simulink model "ex5"  (R2021a)
settings: Solver=VariableStepAuto  StartTime=0.0  StopTime=120  RelTol=1e-7
values from neighbouring files (symbols this model uses):
  a = m*g*l/I    (= 1.96)    [aae666_hw8_ex5.m]
  b = 1/I    (= 0.1)    [aae666_hw8_ex5.m]
  K = [kp kd]    [aae666_hw8_ex5.m]
settings Model: Creator=Tomo  LastModifiedBy=Tomo

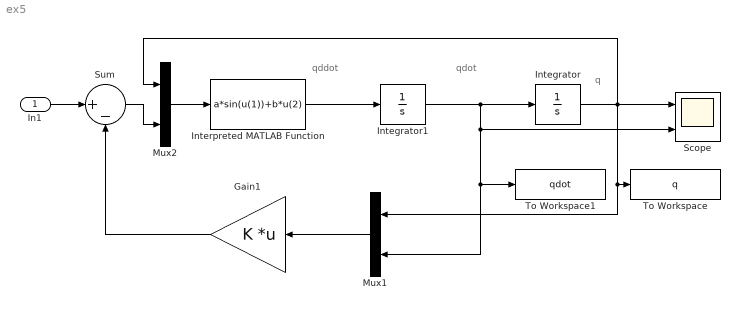
== system ex5 ==
  note: qddot
  note: qdot
  note: q
  In1 : Inport
  Gain1 : Gain  Gain=K  Multiplication=Matrix(K*u)
  Integrator : Integrator  InitialCondition=1
  Integrator1 : Integrator
  Interpreted MATLAB Function : MATLABFcn  MATLABFcn=a*sin(u(1))+b*u(2)
  Mux1 : Mux  Inputs=2
  Mux2 : Mux  Inputs=2
  Scope : Scope  NumInputPorts=2
  Sum : Sum  Inputs=|+-
  To Workspace : ToWorkspace  VariableName=q  SaveFormat=Structure With Time  SampleTime=-1
  To Workspace1 : ToWorkspace  VariableName=qdot  SaveFormat=Structure With Time  SampleTime=-1
  wires:
  Integrator1/1 -> To Workspace1/1, Mux1/2, Scope/2, Integrator/1
  Interpreted MATLAB Function/1 -> Integrator1/1
  Integrator/1 -> Mux2/1, To Workspace/1, Mux1/1, Scope/1
  Gain1/1 -> Sum/2
  Mux1/1 -> Gain1/1
  In1/1 -> Sum/1
  Sum/1 -> Mux2/2
  Mux2/1 -> Interpreted MATLAB Function/1
